simulink model "sim_kinematic_no_steering"  (R2018a)
settings: Solver=ode3  StartTime=0.0  StopTime=10  FixedStep=0.02  RelTol=1e-3
settings Model: Creator=E183308  LastModifiedBy=E183308

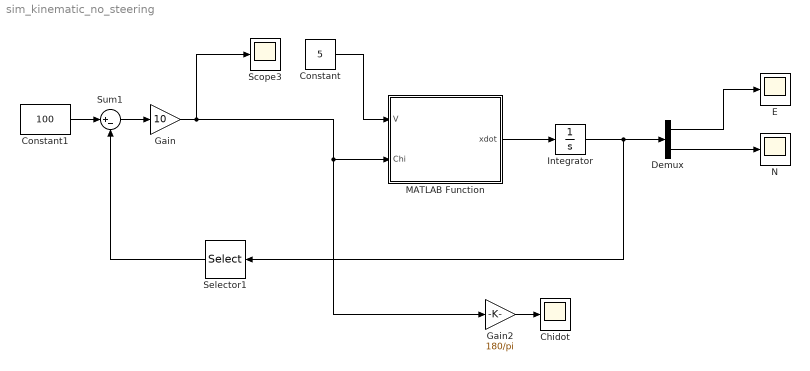
== system sim_kinematic_no_steering ==
  Chidot : Scope
  Constant : Constant  Value=5
  Constant1 : Constant  Value=100
  Demux : Demux  Outputs=2
  E : Scope
  Gain : Gain  Gain=10
  Gain2 : Gain  Gain=180/pi
  Integrator : Integrator  InitialCondition=[0;0]
  MATLAB Function : MATLAB Function  TreatAsAtomicUnit=on
  N : Scope
  Scope3 : Scope
  Selector1 : Selector  InputPortWidth=2  IndexOptions=Index vector (dialog)  Indices=2  OutputSizes=1
  Sum1 : Sum  Inputs=|+-
  wires:
  Sum1/1 -> Gain/1
  Selector1/1 -> Sum1/2
  Constant/1 -> MATLAB Function/1(V)
  MATLAB Function/1(xdot) -> Integrator/1
  Demux/1 -> E/1
  Demux/2 -> N/1
  Integrator/1 -> Selector1/1, Demux/1
  Constant1/1 -> Sum1/1
  Gain2/1 -> Chidot/1
  Gain/1 -> Gain2/1, MATLAB Function/2(Chi), Scope3/1

== matlab function sim_kinematic_no_steering/MATLAB Function ==
  data: xdot output; V input; Chi input
function xdot = kinematic(V,Chi)

Edot = V*sin(Chi);
Ndot = V*cos(Chi);

xdot = [Edot; Ndot];
